simulink model "TrackVehiclesSimulinkExample"  (R2021b)
settings: Solver=FixedStepAuto  StartTime=0.0  StopTime=34.9  FixedStep=0.1  RelTol=1e-3
PreLoadFcn:
  | helperCreateDetectorBus
libraries: motalgorithmslib x1
CloseFcn:
  | % Close opened figure
  | fig = findall(0,'Tag','lidarTrackingExampleDisplay');
  | delete(fig);
settings Model: PauseTimes=15  Creator=The MathWorks, Inc.  LastModifiedBy=ghisl
settings SolverCC: AlgebraicLoopSolver=TrustRegion
settings OptimizationCC: DefaultParameterBehavior=Inlined  EnhancedBackFolding=on  PassReuseOutputArgsThreshold=0  OptimizeBlockOrder=speed  DifferentSizesBufferReuse=on  OptimizationCustomize=off
settings DebuggingCC: ParameterTunabilityLossMsg=error  BusObjectLabelMismatch=error  SymbolicDimsDataTypeCodeGenerationDiagnostic=none  SFMachineParentedDataDiag=warning
settings SFSimCC: MATLABDynamicMemAlloc=off
settings RTWCC: GenerateReport=on  LaunchReport=on
settings CodeAppCC: ForceParamTrailComments=on  OperatorAnnotations=on

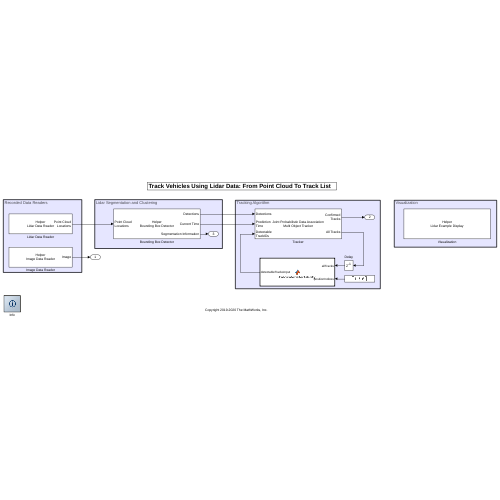
[thumbnail: Simulink's stored preview of the top-level diagram]
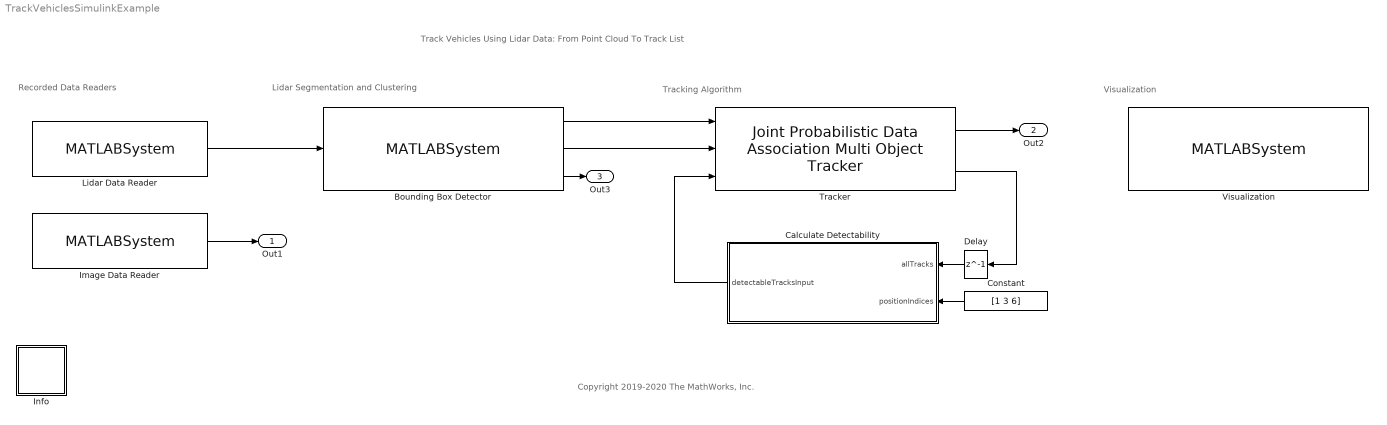
== system TrackVehiclesSimulinkExample ==
  note: Copyright 2019-2020 The MathWorks, Inc.
  note: Visualization
  note: Recorded Data Readers
  note: Tracking Algorithm
  note: Lidar Segmentation and Clustering
  note: Track Vehicles Using Lidar Data: From Point Cloud To Track List
  Bounding Box Detector : MATLABSystem  System=HelperBoundingBoxDetectorBlock  DetectionBusName=detectionBus  SegmentationBusName=segmentationBus  NumLidarPoints=55000  XLimits=[ -70, 70 ]  YLimits=[ -6, 6 ]  ZLimits=[ -2, 10 ]  GroundMaxDistance=0.3  GroundReferenceVector=[ 0, 0, 1 ]  GroundMaxAngularDistance=5  SegmentationMinDistance=1.8  MinDetectionsPerCluster=1  MaxZDistanceCluster=3  MinZDistanceCluster=-3  EgoVehicleRadius=3  MeasurementNoise=blkdiag( 0.25*eye( 3 ), 25, eye( 3 ) )  MeasurementParameters="{  }"  SimulateUsing=Interpreted execution
      mask Type: HelperBoundingBoxDetectorBlock
      mask Display:
      | disp(['Helper' char(10) 'Bounding Box Detector']);
      | port_label('input',1,['Point Cloud' char(10) 'Locations']);
      | port_label('output',1,'Detections');
      | port_label('output',2,'Current Time');
      | port_label('output',3,'Segmentation Information');
  Calculate Detectability : MATLAB Function  TreatAsAtomicUnit=on
  Constant : Constant  Value=[1 3 6]
  Delay : Delay  DelayLength=1
  Image Data Reader : MATLABSystem  System=HelperImageDataReader  TimeStep=0.1  ImageSize=[ 144, 192, 3 ]  ImageFile=imageData_35seconds  ImageDataVariableName=allImageData
      mask Type: HelperImageDataReader
      mask Display:
      | disp(['Helper' char(10) 'Image Data Reader']);
      | port_label('output',1,'Image');
  Info : Subsystem
      settings: OpenFcn=helpview(fullfile(matlabroot,'help','fusion','helptargets.map'),'TrackVehiclesUsingLidarDataInSimulinkExample');
      mask Display: image('demo_info.bmp','center')
  Lidar Data Reader : MATLABSystem  System=HelperLidarDataReader  TimeStep=0.1  NumLidarPoints=55000  LidarFile={ 'lidarData_1', 'lidarData_2', 'lidarData_3', 'lidarData_4', 'lidarData_5' }  LidarDataVariableName=currentLidarData
      mask Type: HelperLidarDataReader
      mask Display:
      | disp(['Helper' char(10) 'Lidar Data Reader']);
      | port_label('output',1,['Point Cloud' char(10) 'Locations']);
  Tracker : motalgorithmslib/Joint Probabilistic Data Association Multi Object Tracker  TrackerIndex=uint32( 0 )  FilterInitializationFcn=helperInitIMMFilter  MaxNumEvents=inf  EventGenerationFcn=jpdaEvents  MaxNumTracks=100  MaxNumSensors=20  TimeTolerance=1e-5  OOSMHandling=Terminate  StateParametersSimulink=struct  HasStateParametersInput=off  SimulateUsing=Interpreted execution  AssignmentThreshold=[75 1000]  InitializationThreshold=0  DetectionProbability=0.9  ClutterDensity=1e-9  TrackLogic=History  pHistoryConfThreshold=[7 10]  pHistoryDelThreshold=[8 10]  pIntegratedConfThreshold=0.95  pIntegratedDelThreshold=0.1  HitMissThreshold=0.1  NewTargetDensity=1e-5  DeathRate=0.01  TimeInputSource=Input port  HasCostMatrixInput=off  HasDetectableTrackIDsInput=on  TentativeTracksOutputPort=off  AllTracksOutputPort=on  InfoOutputPort=off  BusNameSource=Property  BusName=trackBus  BusName2Source=Auto  BusName2=BusTrackerInfo
      settings: SourceProductBaseCode=TF
  Visualization : MATLABSystem  System=HelperLidarExampleDisplayBlock  LidarDataReaderBlockName=Lidar Data Reader  ImageDataReaderBlockName=Image Data Reader  DetectorBlockName=Bounding Box Detector  TrackerBlockName=Tracker  PositionIndex=[ 1, 3, 6 ]  VelocityIndex=[ 2, 4, 7 ]  DimensionIndex=[9 10 11]  YawIndex=8  RecordGIF=true  MovieName=myMovie  SimulateUsing=Interpreted execution
      mask Type: HelperLidarExampleDisplayBlock
      mask Display: disp(['Helper' char(10) 'Lidar Example Display']);
  Out1 : Outport
  Out2 : Outport  Port=2
  Out3 : Outport  Port=3
  wires:
  Constant/1 -> Calculate Detectability/2(positionIndices)
  Delay/1 -> Calculate Detectability/1(allTracks)
  Tracker/2 -> Delay/1
  Lidar Data Reader/1 -> Bounding Box Detector/1
  Calculate Detectability/1(detectableTracksInput) -> Tracker/3
  Image Data Reader/1 -> Out1/1
  Tracker/1 -> Out2/1
  Bounding Box Detector/1 -> Tracker/1
  Bounding Box Detector/2 -> Tracker/2
  Bounding Box Detector/3 -> Out3/1

== system TrackVehiclesSimulinkExample/Info ==

== matlab function TrackVehiclesSimulinkExample/Calculate Detectability ==
  settings: updateMethod=DISCRETE  sampleTime=0.1
  data allTracks settings: description=All Tracks
  data: allTracks input; detectableTracksInput output size=[100 2]; positionIndices input
function detectableTracksInput = CalculateDetectability(allTracks, positionIndices)
% This function calculates the probability of detection for each track. The
% helperCalcDetectability function is used to compute the probability after
% extracting the tracks from the bus.
tracks = allTracks.Tracks(1:allTracks.NumTracks);
detectableTracksInput = helperCalcDetectability(tracks, positionIndices);
end
